simulink model "NeuralcircuitULInjured08102023_DSD"  (R2023a)
settings: Solver=VariableStepAuto  StartTime=0.0  StopTime=1600  RelTol=1e-3
values from neighbouring files (symbols this model uses):
  Cn = 1    [Inhibitory_excitatory_ULInjury_1Hz_08102023.m]    (also in Inhibitory_excitatory_ULInjury_30Hz_08102023.m; InitialExcitatoryInhibitoryNeurons_Healthy08062023.m; InitialExcitatoryInhibitoryULInjured_08102023_DSD.m)
  EK = -84*1    (= -84)    [Inhibitory_excitatory_ULInjury_1Hz_08102023.m]    (also in Inhibitory_excitatory_ULInjury_30Hz_08102023.m; InitialExcitatoryInhibitoryNeurons_Healthy08062023.m; InitialExcitatoryInhibitoryULInjured_08102023_DSD.m)
  EKEx = -90    [Inhibitory_excitatory_ULInjury_1Hz_08102023.m]    (also in Inhibitory_excitatory_ULInjury_30Hz_08102023.m; InitialExcitatoryInhibitoryNeurons_Healthy08062023.m; InitialExcitatoryInhibitoryULInjured_08102023_DSD.m)
  EKIn = -90    [Inhibitory_excitatory_ULInjury_1Hz_08102023.m]    (also in Inhibitory_excitatory_ULInjury_30Hz_08102023.m; InitialExcitatoryInhibitoryNeurons_Healthy08062023.m; InitialExcitatoryInhibitoryULInjured_08102023_DSD.m)
  ELEx = -65    [Inhibitory_excitatory_ULInjury_1Hz_08102023.m]    (also in Inhibitory_excitatory_ULInjury_30Hz_08102023.m; InitialExcitatoryInhibitoryNeurons_Healthy08062023.m; InitialExcitatoryInhibitoryULInjured_08102023_DSD.m)
  ELIn = -65    [Inhibitory_excitatory_ULInjury_1Hz_08102023.m]    (also in Inhibitory_excitatory_ULInjury_30Hz_08102023.m; InitialExcitatoryInhibitoryNeurons_Healthy08062023.m; InitialExcitatoryInhibitoryULInjured_08102023_DSD.m)
  ELk = -83.38*1    (= -83.38)    [Inhibitory_excitatory_ULInjury_1Hz_08102023.m]    (also in Inhibitory_excitatory_ULInjury_30Hz_08102023.m; InitialExcitatoryInhibitoryNeurons_Healthy08062023.m; InitialExcitatoryInhibitoryULInjured_08102023_DSD.m)
  ENa = 50*1    (= 50)    [Inhibitory_excitatory_ULInjury_1Hz_08102023.m]    (also in Inhibitory_excitatory_ULInjury_30Hz_08102023.m; InitialExcitatoryInhibitoryNeurons_Healthy08062023.m; InitialExcitatoryInhibitoryULInjured_08102023_DSD.m)
  ENaEx = 60    [Inhibitory_excitatory_ULInjury_1Hz_08102023.m]    (also in Inhibitory_excitatory_ULInjury_30Hz_08102023.m; InitialExcitatoryInhibitoryNeurons_Healthy08062023.m; InitialExcitatoryInhibitoryULInjured_08102023_DSD.m)
  ENaIn = 55    [Inhibitory_excitatory_ULInjury_1Hz_08102023.m]    (also in Inhibitory_excitatory_ULInjury_30Hz_08102023.m; InitialExcitatoryInhibitoryNeurons_Healthy08062023.m; InitialExcitatoryInhibitoryULInjured_08102023_DSD.m)
  ErestE = -65    [Inhibitory_excitatory_ULInjury_1Hz_08102023.m]    (also in Inhibitory_excitatory_ULInjury_30Hz_08102023.m; InitialExcitatoryInhibitoryNeurons_Healthy08062023.m; InitialExcitatoryInhibitoryULInjured_08102023_DSD.m)
  ErestIn = -64    [Inhibitory_excitatory_ULInjury_1Hz_08102023.m]    (also in Inhibitory_excitatory_ULInjury_30Hz_08102023.m; InitialExcitatoryInhibitoryNeurons_Healthy08062023.m; InitialExcitatoryInhibitoryULInjured_08102023_DSD.m)
  ESynE = -10    [Inhibitory_excitatory_ULInjury_1Hz_08102023.m]    (also in Inhibitory_excitatory_ULInjury_30Hz_08102023.m; InitialExcitatoryInhibitoryNeurons_Healthy08062023.m; InitialExcitatoryInhibitoryULInjured_08102023_DSD.m)
  ESynE2 = -10    [Inhibitory_excitatory_ULInjury_1Hz_08102023.m]    (also in Inhibitory_excitatory_ULInjury_30Hz_08102023.m; InitialExcitatoryInhibitoryNeurons_Healthy08062023.m; InitialExcitatoryInhibitoryULInjured_08102023_DSD.m)
  ESynE3 = -10    [Inhibitory_excitatory_ULInjury_1Hz_08102023.m]    (also in Inhibitory_excitatory_ULInjury_30Hz_08102023.m; InitialExcitatoryInhibitoryNeurons_Healthy08062023.m; InitialExcitatoryInhibitoryULInjured_08102023_DSD.m)
  ESynE4 = -10    [Inhibitory_excitatory_ULInjury_1Hz_08102023.m]    (also in Inhibitory_excitatory_ULInjury_30Hz_08102023.m; InitialExcitatoryInhibitoryNeurons_Healthy08062023.m; InitialExcitatoryInhibitoryULInjured_08102023_DSD.m)
  ESynE5 = -10    [Inhibitory_excitatory_ULInjury_1Hz_08102023.m]    (also in Inhibitory_excitatory_ULInjury_30Hz_08102023.m; InitialExcitatoryInhibitoryNeurons_Healthy08062023.m; InitialExcitatoryInhibitoryULInjured_08102023_DSD.m)
  ESynE6 = -15    [Inhibitory_excitatory_ULInjury_1Hz_08102023.m]    (also in Inhibitory_excitatory_ULInjury_30Hz_08102023.m; InitialExcitatoryInhibitoryNeurons_Healthy08062023.m; InitialExcitatoryInhibitoryULInjured_08102023_DSD.m = -10)
  ESynE7 = -10    [Inhibitory_excitatory_ULInjury_1Hz_08102023.m]    (also in Inhibitory_excitatory_ULInjury_30Hz_08102023.m; InitialExcitatoryInhibitoryNeurons_Healthy08062023.m; InitialExcitatoryInhibitoryULInjured_08102023_DSD.m)
  ESynI = -80    [Inhibitory_excitatory_ULInjury_1Hz_08102023.m]    (also in Inhibitory_excitatory_ULInjury_30Hz_08102023.m; InitialExcitatoryInhibitoryNeurons_Healthy08062023.m; InitialExcitatoryInhibitoryULInjured_08102023_DSD.m)
  ESynI2 = -80    [Inhibitory_excitatory_ULInjury_1Hz_08102023.m]    (also in Inhibitory_excitatory_ULInjury_30Hz_08102023.m; InitialExcitatoryInhibitoryNeurons_Healthy08062023.m; InitialExcitatoryInhibitoryULInjured_08102023_DSD.m)
  ESynI3 = -80    [Inhibitory_excitatory_ULInjury_1Hz_08102023.m]    (also in Inhibitory_excitatory_ULInjury_30Hz_08102023.m; InitialExcitatoryInhibitoryNeurons_Healthy08062023.m; InitialExcitatoryInhibitoryULInjured_08102023_DSD.m)
  ESynI5 = -80    [Inhibitory_excitatory_ULInjury_1Hz_08102023.m]    (also in Inhibitory_excitatory_ULInjury_30Hz_08102023.m; InitialExcitatoryInhibitoryNeurons_Healthy08062023.m; InitialExcitatoryInhibitoryULInjured_08102023_DSD.m)
  ESynI6 = -65    [Inhibitory_excitatory_ULInjury_1Hz_08102023.m]    (also in Inhibitory_excitatory_ULInjury_30Hz_08102023.m; InitialExcitatoryInhibitoryNeurons_Healthy08062023.m; InitialExcitatoryInhibitoryULInjured_08102023_DSD.m = -80)
  Exh0 = ahEx(V0)./(ahEx(V0)+bhEx(V0))    [Inhibitory_excitatory_ULInjury_1Hz_08102023.m]    (also in Inhibitory_excitatory_ULInjury_30Hz_08102023.m; InitialExcitatoryInhibitoryNeurons_Healthy08062023.m; InitialExcitatoryInhibitoryULInjured_08102023_DSD.m)
  Exm0 = amEx(V0)./(amEx(V0)+bmEx(V0))    [Inhibitory_excitatory_ULInjury_1Hz_08102023.m]    (also in Inhibitory_excitatory_ULInjury_30Hz_08102023.m; InitialExcitatoryInhibitoryNeurons_Healthy08062023.m; InitialExcitatoryInhibitoryULInjured_08102023_DSD.m)
  Exn0 = anEx(V0)./(anEx(V0)+bnEx(V0))    [Inhibitory_excitatory_ULInjury_1Hz_08102023.m]    (also in Inhibitory_excitatory_ULInjury_30Hz_08102023.m; InitialExcitatoryInhibitoryNeurons_Healthy08062023.m; InitialExcitatoryInhibitoryULInjured_08102023_DSD.m)
  Ga = 1*Gaxial    (= 0.351233961271)    [Inhibitory_excitatory_ULInjury_1Hz_08102023.m]    (also in Inhibitory_excitatory_ULInjury_30Hz_08102023.m; InitialExcitatoryInhibitoryNeurons_Healthy08062023.m; InitialExcitatoryInhibitoryULInjured_08102023_DSD.m)
  Gaxial = pi*(d^2)/(4*Ro_ax*Internodal_L)*1e7    (= 0.351233961271)    [Inhibitory_excitatory_ULInjury_1Hz_08102023.m]    (also in Inhibitory_excitatory_ULInjury_30Hz_08102023.m; InitialExcitatoryInhibitoryNeurons_Healthy08062023.m; InitialExcitatoryInhibitoryULInjured_08102023_DSD.m)
  gKEx = 100    [Inhibitory_excitatory_ULInjury_1Hz_08102023.m]    (also in Inhibitory_excitatory_ULInjury_30Hz_08102023.m; InitialExcitatoryInhibitoryNeurons_Healthy08062023.m; InitialExcitatoryInhibitoryULInjured_08102023_DSD.m)
  gKIn = 9    [Inhibitory_excitatory_ULInjury_1Hz_08102023.m]    (also in Inhibitory_excitatory_ULInjury_30Hz_08102023.m; InitialExcitatoryInhibitoryNeurons_Healthy08062023.m; InitialExcitatoryInhibitoryULInjured_08102023_DSD.m)
  gKs = 10*0.08/1    (= 0.8)    [Inhibitory_excitatory_ULInjury_1Hz_08102023.m]    (also in Inhibitory_excitatory_ULInjury_30Hz_08102023.m; InitialExcitatoryInhibitoryNeurons_Healthy08062023.m; InitialExcitatoryInhibitoryULInjured_08102023_DSD.m)
  gLEx = 0.1    [Inhibitory_excitatory_ULInjury_1Hz_08102023.m]    (also in Inhibitory_excitatory_ULInjury_30Hz_08102023.m; InitialExcitatoryInhibitoryNeurons_Healthy08062023.m; InitialExcitatoryInhibitoryULInjured_08102023_DSD.m)
  gLIn = 0.1    [Inhibitory_excitatory_ULInjury_1Hz_08102023.m]    (also in Inhibitory_excitatory_ULInjury_30Hz_08102023.m; InitialExcitatoryInhibitoryNeurons_Healthy08062023.m; InitialExcitatoryInhibitoryULInjured_08102023_DSD.m)
  gLk = 10*0.08/1    (= 0.8)    [Inhibitory_excitatory_ULInjury_1Hz_08102023.m]    (also in Inhibitory_excitatory_ULInjury_30Hz_08102023.m; InitialExcitatoryInhibitoryNeurons_Healthy08062023.m; InitialExcitatoryInhibitoryULInjured_08102023_DSD.m)
  gNaEx = 30    [Inhibitory_excitatory_ULInjury_1Hz_08102023.m]    (also in Inhibitory_excitatory_ULInjury_30Hz_08102023.m; InitialExcitatoryInhibitoryNeurons_Healthy08062023.m; InitialExcitatoryInhibitoryULInjured_08102023_DSD.m)
  gNaf = 10*3/1    (= 30)    [Inhibitory_excitatory_ULInjury_1Hz_08102023.m]    (also in Inhibitory_excitatory_ULInjury_30Hz_08102023.m; InitialExcitatoryInhibitoryNeurons_Healthy08062023.m; InitialExcitatoryInhibitoryULInjured_08102023_DSD.m)
  gNaIn = 35    [Inhibitory_excitatory_ULInjury_1Hz_08102023.m]    (also in Inhibitory_excitatory_ULInjury_30Hz_08102023.m; InitialExcitatoryInhibitoryNeurons_Healthy08062023.m; InitialExcitatoryInhibitoryULInjured_08102023_DSD.m)
  gNap = 10*0.005/1    (= 0.05)    [Inhibitory_excitatory_ULInjury_1Hz_08102023.m]    (also in Inhibitory_excitatory_ULInjury_30Hz_08102023.m; InitialExcitatoryInhibitoryNeurons_Healthy08062023.m; InitialExcitatoryInhibitoryULInjured_08102023_DSD.m)
  gSynE = 0.08    [Inhibitory_excitatory_ULInjury_1Hz_08102023.m]    (also in Inhibitory_excitatory_ULInjury_30Hz_08102023.m; InitialExcitatoryInhibitoryNeurons_Healthy08062023.m; InitialExcitatoryInhibitoryULInjured_08102023_DSD.m)
  gSynE2 = 0.08    [Inhibitory_excitatory_ULInjury_1Hz_08102023.m]    (also in Inhibitory_excitatory_ULInjury_30Hz_08102023.m; InitialExcitatoryInhibitoryNeurons_Healthy08062023.m; InitialExcitatoryInhibitoryULInjured_08102023_DSD.m)
  gSynE3 = 0.08    [Inhibitory_excitatory_ULInjury_1Hz_08102023.m]    (also in Inhibitory_excitatory_ULInjury_30Hz_08102023.m; InitialExcitatoryInhibitoryNeurons_Healthy08062023.m; InitialExcitatoryInhibitoryULInjured_08102023_DSD.m)
  gSynE4 = 0.08    [Inhibitory_excitatory_ULInjury_1Hz_08102023.m]    (also in Inhibitory_excitatory_ULInjury_30Hz_08102023.m; InitialExcitatoryInhibitoryNeurons_Healthy08062023.m; InitialExcitatoryInhibitoryULInjured_08102023_DSD.m)
  gSynE5 = 0.08    [Inhibitory_excitatory_ULInjury_1Hz_08102023.m]    (also in Inhibitory_excitatory_ULInjury_30Hz_08102023.m; InitialExcitatoryInhibitoryNeurons_Healthy08062023.m; InitialExcitatoryInhibitoryULInjured_08102023_DSD.m)
  gSynE6 = 0.08    [Inhibitory_excitatory_ULInjury_1Hz_08102023.m]    (also in Inhibitory_excitatory_ULInjury_30Hz_08102023.m; InitialExcitatoryInhibitoryNeurons_Healthy08062023.m; InitialExcitatoryInhibitoryULInjured_08102023_DSD.m)
  gSynE7 = 0.165    [Inhibitory_excitatory_ULInjury_1Hz_08102023.m]    (also in Inhibitory_excitatory_ULInjury_30Hz_08102023.m; InitialExcitatoryInhibitoryNeurons_Healthy08062023.m; InitialExcitatoryInhibitoryULInjured_08102023_DSD.m)
  gSynI = 0.8    [Inhibitory_excitatory_ULInjury_1Hz_08102023.m]    (also in Inhibitory_excitatory_ULInjury_30Hz_08102023.m; InitialExcitatoryInhibitoryNeurons_Healthy08062023.m; InitialExcitatoryInhibitoryULInjured_08102023_DSD.m)
  gSynI2 = 0.12    [Inhibitory_excitatory_ULInjury_1Hz_08102023.m]    (also in Inhibitory_excitatory_ULInjury_30Hz_08102023.m; InitialExcitatoryInhibitoryNeurons_Healthy08062023.m; InitialExcitatoryInhibitoryULInjured_08102023_DSD.m)
  gSynI3 = 0.12    [Inhibitory_excitatory_ULInjury_1Hz_08102023.m]    (also in Inhibitory_excitatory_ULInjury_30Hz_08102023.m; InitialExcitatoryInhibitoryNeurons_Healthy08062023.m; InitialExcitatoryInhibitoryULInjured_08102023_DSD.m)
  gSynI5 = 0.12    [Inhibitory_excitatory_ULInjury_1Hz_08102023.m]    (also in Inhibitory_excitatory_ULInjury_30Hz_08102023.m; InitialExcitatoryInhibitoryNeurons_Healthy08062023.m; InitialExcitatoryInhibitoryULInjured_08102023_DSD.m)
  gSynI6 = 0.12    [Inhibitory_excitatory_ULInjury_1Hz_08102023.m]    (also in Inhibitory_excitatory_ULInjury_30Hz_08102023.m; InitialExcitatoryInhibitoryNeurons_Healthy08062023.m; InitialExcitatoryInhibitoryULInjured_08102023_DSD.m)
  h0 = ah(V0O)./(ah(V0O)+bh(V0O))    [Inhibitory_excitatory_ULInjury_1Hz_08102023.m]    (also in Inhibitory_excitatory_ULInjury_30Hz_08102023.m; InitialExcitatoryInhibitoryNeurons_Healthy08062023.m; InitialExcitatoryInhibitoryULInjured_08102023_DSD.m)
  Inh0 = ahIn(ErestIn)./(ahIn(ErestIn)+bhIn(ErestIn))    [Inhibitory_excitatory_ULInjury_1Hz_08102023.m]    (also in Inhibitory_excitatory_ULInjury_30Hz_08102023.m; InitialExcitatoryInhibitoryNeurons_Healthy08062023.m; InitialExcitatoryInhibitoryULInjured_08102023_DSD.m)
  Inm0 = amIn(ErestIn)./(amIn(ErestIn)+bmIn(ErestIn))    [Inhibitory_excitatory_ULInjury_1Hz_08102023.m]    (also in Inhibitory_excitatory_ULInjury_30Hz_08102023.m; InitialExcitatoryInhibitoryNeurons_Healthy08062023.m; InitialExcitatoryInhibitoryULInjured_08102023_DSD.m)
  Inn0 = anIn(ErestIn)./(anIn(ErestIn)+bnIn(ErestIn))    [Inhibitory_excitatory_ULInjury_1Hz_08102023.m]    (also in Inhibitory_excitatory_ULInjury_30Hz_08102023.m; InitialExcitatoryInhibitoryNeurons_Healthy08062023.m; InitialExcitatoryInhibitoryULInjured_08102023_DSD.m)
  m0 = am(V0O)./(am(V0O)+Bm(V0O))    [Inhibitory_excitatory_ULInjury_1Hz_08102023.m]    (also in Inhibitory_excitatory_ULInjury_30Hz_08102023.m; InitialExcitatoryInhibitoryNeurons_Healthy08062023.m; InitialExcitatoryInhibitoryULInjured_08102023_DSD.m)
  mNap0 = amNap(V0)./(amNap(V0O)+bmNap(V0O))    [Inhibitory_excitatory_ULInjury_1Hz_08102023.m]    (also in Inhibitory_excitatory_ULInjury_30Hz_08102023.m; InitialExcitatoryInhibitoryNeurons_Healthy08062023.m; InitialExcitatoryInhibitoryULInjured_08102023_DSD.m)
  Ro_e = 500    [Inhibitory_excitatory_ULInjury_1Hz_08102023.m]    (also in Inhibitory_excitatory_ULInjury_30Hz_08102023.m; InitialExcitatoryInhibitoryNeurons_Healthy08062023.m; InitialExcitatoryInhibitoryULInjured_08102023_DSD.m)
  s0 = as(V0O)./(as(V0O)+bs(V0O))    [Inhibitory_excitatory_ULInjury_1Hz_08102023.m]    (also in Inhibitory_excitatory_ULInjury_30Hz_08102023.m; InitialExcitatoryInhibitoryNeurons_Healthy08062023.m; InitialExcitatoryInhibitoryULInjured_08102023_DSD.m)
  TawIExt = 30    [Inhibitory_excitatory_ULInjury_1Hz_08102023.m]    (also in Inhibitory_excitatory_ULInjury_30Hz_08102023.m; InitialExcitatoryInhibitoryNeurons_Healthy08062023.m = 200; InitialExcitatoryInhibitoryULInjured_08102023_DSD.m = 200)
  TawIExtE = 30    [Inhibitory_excitatory_ULInjury_1Hz_08102023.m]    (also in Inhibitory_excitatory_ULInjury_30Hz_08102023.m; InitialExcitatoryInhibitoryNeurons_Healthy08062023.m = 1; InitialExcitatoryInhibitoryULInjured_08102023_DSD.m = 10)
  TawSynE = 5    [Inhibitory_excitatory_ULInjury_1Hz_08102023.m]    (also in Inhibitory_excitatory_ULInjury_30Hz_08102023.m; InitialExcitatoryInhibitoryNeurons_Healthy08062023.m; InitialExcitatoryInhibitoryULInjured_08102023_DSD.m)
  TawSynE2 = 11    [Inhibitory_excitatory_ULInjury_1Hz_08102023.m]    (also in Inhibitory_excitatory_ULInjury_30Hz_08102023.m; InitialExcitatoryInhibitoryNeurons_Healthy08062023.m = 12; InitialExcitatoryInhibitoryULInjured_08102023_DSD.m = 5)
  TawSynE3 = 10    [Inhibitory_excitatory_ULInjury_1Hz_08102023.m]    (also in Inhibitory_excitatory_ULInjury_30Hz_08102023.m; InitialExcitatoryInhibitoryNeurons_Healthy08062023.m = 18; InitialExcitatoryInhibitoryULInjured_08102023_DSD.m = 8)
  TawSynE4 = 6    [Inhibitory_excitatory_ULInjury_1Hz_08102023.m]    (also in Inhibitory_excitatory_ULInjury_30Hz_08102023.m; InitialExcitatoryInhibitoryNeurons_Healthy08062023.m; InitialExcitatoryInhibitoryULInjured_08102023_DSD.m)
  TawSynE41 = 14    [Inhibitory_excitatory_ULInjury_1Hz_08102023.m]    (also in Inhibitory_excitatory_ULInjury_30Hz_08102023.m; InitialExcitatoryInhibitoryNeurons_Healthy08062023.m = 15; InitialExcitatoryInhibitoryULInjured_08102023_DSD.m = 6)
  TawSynE5 = 6    [Inhibitory_excitatory_ULInjury_1Hz_08102023.m]    (also in Inhibitory_excitatory_ULInjury_30Hz_08102023.m; InitialExcitatoryInhibitoryNeurons_Healthy08062023.m; InitialExcitatoryInhibitoryULInjured_08102023_DSD.m)
  TawSynE6 = 3    [Inhibitory_excitatory_ULInjury_1Hz_08102023.m]    (also in Inhibitory_excitatory_ULInjury_30Hz_08102023.m; InitialExcitatoryInhibitoryNeurons_Healthy08062023.m; InitialExcitatoryInhibitoryULInjured_08102023_DSD.m)
  TawSynE66 = 1    [Inhibitory_excitatory_ULInjury_1Hz_08102023.m]    (also in Inhibitory_excitatory_ULInjury_30Hz_08102023.m; InitialExcitatoryInhibitoryNeurons_Healthy08062023.m; InitialExcitatoryInhibitoryULInjured_08102023_DSD.m)
  TawSynE66E = 5    [Inhibitory_excitatory_ULInjury_1Hz_08102023.m]    (also in Inhibitory_excitatory_ULInjury_30Hz_08102023.m; InitialExcitatoryInhibitoryNeurons_Healthy08062023.m; InitialExcitatoryInhibitoryULInjured_08102023_DSD.m)
  TawSynE7 = 0.05    [Inhibitory_excitatory_ULInjury_1Hz_08102023.m]    (also in Inhibitory_excitatory_ULInjury_30Hz_08102023.m; InitialExcitatoryInhibitoryNeurons_Healthy08062023.m; InitialExcitatoryInhibitoryULInjured_08102023_DSD.m)
  TawSynI = 5    [Inhibitory_excitatory_ULInjury_1Hz_08102023.m]    (also in Inhibitory_excitatory_ULInjury_30Hz_08102023.m; InitialExcitatoryInhibitoryNeurons_Healthy08062023.m; InitialExcitatoryInhibitoryULInjured_08102023_DSD.m)
  TawSynI2 = 1    [Inhibitory_excitatory_ULInjury_1Hz_08102023.m]    (also in Inhibitory_excitatory_ULInjury_30Hz_08102023.m; InitialExcitatoryInhibitoryNeurons_Healthy08062023.m; InitialExcitatoryInhibitoryULInjured_08102023_DSD.m = 2)
  TawSynI3 = 30    [Inhibitory_excitatory_ULInjury_1Hz_08102023.m]    (also in Inhibitory_excitatory_ULInjury_30Hz_08102023.m; InitialExcitatoryInhibitoryNeurons_Healthy08062023.m = 35; InitialExcitatoryInhibitoryULInjured_08102023_DSD.m)
  TawSynI5 = 4    [Inhibitory_excitatory_ULInjury_1Hz_08102023.m]    (also in Inhibitory_excitatory_ULInjury_30Hz_08102023.m; InitialExcitatoryInhibitoryNeurons_Healthy08062023.m = 1; InitialExcitatoryInhibitoryULInjured_08102023_DSD.m = 1)
  TawSynI6 = 3    [Inhibitory_excitatory_ULInjury_1Hz_08102023.m]    (also in Inhibitory_excitatory_ULInjury_30Hz_08102023.m; InitialExcitatoryInhibitoryNeurons_Healthy08062023.m; InitialExcitatoryInhibitoryULInjured_08102023_DSD.m)
  TawSynI7 = 0.01    [Inhibitory_excitatory_ULInjury_1Hz_08102023.m]    (also in Inhibitory_excitatory_ULInjury_30Hz_08102023.m; InitialExcitatoryInhibitoryNeurons_Healthy08062023.m; InitialExcitatoryInhibitoryULInjured_08102023_DSD.m)
  V0 = -65    [Inhibitory_excitatory_ULInjury_1Hz_08102023.m]    (also in Inhibitory_excitatory_ULInjury_30Hz_08102023.m; InitialExcitatoryInhibitoryNeurons_Healthy08062023.m; InitialExcitatoryInhibitoryULInjured_08102023_DSD.m)
  V0In = -64    [Inhibitory_excitatory_ULInjury_1Hz_08102023.m]    (also in Inhibitory_excitatory_ULInjury_30Hz_08102023.m; InitialExcitatoryInhibitoryNeurons_Healthy08062023.m; InitialExcitatoryInhibitoryULInjured_08102023_DSD.m)
  w12 = -0.2    [Inhibitory_excitatory_ULInjury_1Hz_08102023.m]    (also in Inhibitory_excitatory_ULInjury_30Hz_08102023.m; InitialExcitatoryInhibitoryNeurons_Healthy08062023.m = -0.28; InitialExcitatoryInhibitoryULInjured_08102023_DSD.m = -0.35)
  w14 = 0.05    [Inhibitory_excitatory_ULInjury_1Hz_08102023.m]    (also in Inhibitory_excitatory_ULInjury_30Hz_08102023.m; InitialExcitatoryInhibitoryNeurons_Healthy08062023.m = 0.09; InitialExcitatoryInhibitoryULInjured_08102023_DSD.m = 0.09)
  w15 = -0.45    [Inhibitory_excitatory_ULInjury_1Hz_08102023.m]    (also in Inhibitory_excitatory_ULInjury_30Hz_08102023.m = -0.07; InitialExcitatoryInhibitoryNeurons_Healthy08062023.m = -0.4; InitialExcitatoryInhibitoryULInjured_08102023_DSD.m = -0.4)
  w17 = -0.25    [Inhibitory_excitatory_ULInjury_1Hz_08102023.m]    (also in Inhibitory_excitatory_ULInjury_30Hz_08102023.m; InitialExcitatoryInhibitoryNeurons_Healthy08062023.m; InitialExcitatoryInhibitoryULInjured_08102023_DSD.m)
  w26 = 0.2    [Inhibitory_excitatory_ULInjury_1Hz_08102023.m]    (also in Inhibitory_excitatory_ULInjury_30Hz_08102023.m = 0.25; InitialExcitatoryInhibitoryNeurons_Healthy08062023.m = 0.05; InitialExcitatoryInhibitoryULInjured_08102023_DSD.m = 0.05)
  w28 = 0.165    [Inhibitory_excitatory_ULInjury_1Hz_08102023.m]    (also in Inhibitory_excitatory_ULInjury_30Hz_08102023.m; InitialExcitatoryInhibitoryNeurons_Healthy08062023.m = 0.13; InitialExcitatoryInhibitoryULInjured_08102023_DSD.m = 0.13)
  w34 = 0.09    [Inhibitory_excitatory_ULInjury_1Hz_08102023.m]    (also in Inhibitory_excitatory_ULInjury_30Hz_08102023.m; InitialExcitatoryInhibitoryNeurons_Healthy08062023.m = 0.03; InitialExcitatoryInhibitoryULInjured_08102023_DSD.m = 0.06)
  w63 = -0.12    [Inhibitory_excitatory_ULInjury_1Hz_08102023.m]    (also in Inhibitory_excitatory_ULInjury_30Hz_08102023.m; InitialExcitatoryInhibitoryNeurons_Healthy08062023.m = -0.08; InitialExcitatoryInhibitoryULInjured_08102023_DSD.m = -0.27)
  w66 = 0.03    [Inhibitory_excitatory_ULInjury_1Hz_08102023.m]    (also in Inhibitory_excitatory_ULInjury_30Hz_08102023.m; InitialExcitatoryInhibitoryNeurons_Healthy08062023.m; InitialExcitatoryInhibitoryULInjured_08102023_DSD.m)
  w66E = 0.2    [Inhibitory_excitatory_ULInjury_1Hz_08102023.m]    (also in Inhibitory_excitatory_ULInjury_30Hz_08102023.m; InitialExcitatoryInhibitoryNeurons_Healthy08062023.m = 0.09; InitialExcitatoryInhibitoryULInjured_08102023_DSD.m = 0.1)
  w67 = -0.4    [Inhibitory_excitatory_ULInjury_1Hz_08102023.m]    (also in Inhibitory_excitatory_ULInjury_30Hz_08102023.m; InitialExcitatoryInhibitoryNeurons_Healthy08062023.m = -0.55; InitialExcitatoryInhibitoryULInjured_08102023_DSD.m = -0.55)
  w68 = 0.35    [Inhibitory_excitatory_ULInjury_1Hz_08102023.m]    (also in Inhibitory_excitatory_ULInjury_30Hz_08102023.m; InitialExcitatoryInhibitoryNeurons_Healthy08062023.m = 0.1; InitialExcitatoryInhibitoryULInjured_08102023_DSD.m = 0.1)
  w71 = 0.25    [Inhibitory_excitatory_ULInjury_1Hz_08102023.m]    (also in Inhibitory_excitatory_ULInjury_30Hz_08102023.m; InitialExcitatoryInhibitoryNeurons_Healthy08062023.m; InitialExcitatoryInhibitoryULInjured_08102023_DSD.m)
  w78 = 0.25    [Inhibitory_excitatory_ULInjury_1Hz_08102023.m]    (also in Inhibitory_excitatory_ULInjury_30Hz_08102023.m; InitialExcitatoryInhibitoryNeurons_Healthy08062023.m; InitialExcitatoryInhibitoryULInjured_08102023_DSD.m)
  w79 = 0.35    [Inhibitory_excitatory_ULInjury_1Hz_08102023.m]    (also in Inhibitory_excitatory_ULInjury_30Hz_08102023.m; InitialExcitatoryInhibitoryNeurons_Healthy08062023.m; InitialExcitatoryInhibitoryULInjured_08102023_DSD.m)
  w83 = 0.2    [Inhibitory_excitatory_ULInjury_1Hz_08102023.m]    (also in Inhibitory_excitatory_ULInjury_30Hz_08102023.m; InitialExcitatoryInhibitoryNeurons_Healthy08062023.m = 0.13; InitialExcitatoryInhibitoryULInjured_08102023_DSD.m = 0.08)
  w85 = 0.1    [Inhibitory_excitatory_ULInjury_1Hz_08102023.m]    (also in Inhibitory_excitatory_ULInjury_30Hz_08102023.m = 0.12; InitialExcitatoryInhibitoryNeurons_Healthy08062023.m = 0.04; InitialExcitatoryInhibitoryULInjured_08102023_DSD.m = 0.05)
  X = nan(node,1)    [Inhibitory_excitatory_ULInjury_1Hz_08102023.m]    (also in Inhibitory_excitatory_ULInjury_30Hz_08102023.m; InitialExcitatoryInhibitoryNeurons_Healthy08062023.m; InitialExcitatoryInhibitoryULInjured_08102023_DSD.m)
  X2 = nan(node2,1)    [Inhibitory_excitatory_ULInjury_1Hz_08102023.m]    (also in Inhibitory_excitatory_ULInjury_30Hz_08102023.m; InitialExcitatoryInhibitoryNeurons_Healthy08062023.m; InitialExcitatoryInhibitoryULInjured_08102023_DSD.m)
  Xelec = Xtotal-Nodal_L*9-Internodal_L*9    (= 0.1152)    [Inhibitory_excitatory_ULInjury_1Hz_08102023.m]    (also in Inhibitory_excitatory_ULInjury_30Hz_08102023.m; InitialExcitatoryInhibitoryNeurons_Healthy08062023.m; InitialExcitatoryInhibitoryULInjured_08102023_DSD.m)
  Xelec2 = 1/(10000)+Nodal_L2*(node2-1)/2+Internodal_L2*(node2-1)/2    (= 0.0001)    [Inhibitory_excitatory_ULInjury_1Hz_08102023.m]    (also in Inhibitory_excitatory_ULInjury_30Hz_08102023.m; InitialExcitatoryInhibitoryNeurons_Healthy08062023.m; InitialExcitatoryInhibitoryULInjured_08102023_DSD.m)
  Y = nan(node,1)    [Inhibitory_excitatory_ULInjury_1Hz_08102023.m]    (also in Inhibitory_excitatory_ULInjury_30Hz_08102023.m; InitialExcitatoryInhibitoryNeurons_Healthy08062023.m; InitialExcitatoryInhibitoryULInjured_08102023_DSD.m)
  Y2 = nan(node2,1)    [Inhibitory_excitatory_ULInjury_1Hz_08102023.m]    (also in Inhibitory_excitatory_ULInjury_30Hz_08102023.m; InitialExcitatoryInhibitoryNeurons_Healthy08062023.m; InitialExcitatoryInhibitoryULInjured_08102023_DSD.m)
  Yelec = 100/10000    (= 0.01)    [Inhibitory_excitatory_ULInjury_1Hz_08102023.m]    (also in Inhibitory_excitatory_ULInjury_30Hz_08102023.m; InitialExcitatoryInhibitoryNeurons_Healthy08062023.m; InitialExcitatoryInhibitoryULInjured_08102023_DSD.m)
  Yelec2 = 500/10000    (= 0.05)    [Inhibitory_excitatory_ULInjury_1Hz_08102023.m]    (also in Inhibitory_excitatory_ULInjury_30Hz_08102023.m; InitialExcitatoryInhibitoryNeurons_Healthy08062023.m; InitialExcitatoryInhibitoryULInjured_08102023_DSD.m)
libraries: simulink x1
(part 13 of 14)

== system NeuralcircuitULInjured08102023_DSD/Neuron 8/Node 6/Naf/h ==
  Vi : Inport
  Add : Sum  Inputs=+-
  Add1 : Sum
  Add2 : Sum  Inputs=+-
  Add3 : Sum  Inputs=+-
  Add4 : Sum
  Add5 : Sum
  Beta_h : Product  Inputs=*/
  Constant : Constant
  Constant1 : Constant  Value=0.0336
  Constant10 : Constant  Value=13.4
  Constant2 : Constant  Value=118
  Constant3 : Constant
  Constant5 : Constant  Value=11
  Constant6 : Constant  Value=2.3
  Constant7 : Constant  Value=35.8
  Constant8 : Constant
  Divide : Product  Inputs=**
  Divide1 : Product  Inputs=**
  Divide4 : Product  Inputs=*/
  Divide5 : Product  Inputs=**
  Divide6 : Product  Inputs=*/
  Gain : Gain  Gain=-1
  Gain1 : Gain  Gain=-1
  Integrator Limited : Integrator  InitialCondition=h0  UpperSaturationLimit=1  LowerSaturationLimit=0
  Math Function : Math  SignedPower=on
  Math Function1 : Math  SignedPower=on
  alpha_h1 : Product  Inputs=*/
  hNaf : Outport  VectorParamsAs1DForOutWhenUnconnected=off
  wires:
  Add5/1 -> Beta_h/2
  Divide/1 -> Add3/1
  Constant6/1 -> Beta_h/1
  Divide5/1 -> Add3/2
  Add/1 -> Divide/1
  Constant/1 -> Add/1
  Add1/1 -> Divide4/1, Gain1/1
  Constant2/1 -> Add1/1
  Constant7/1 -> Add4/1
  Constant8/1 -> Add5/1
  Add4/1 -> Gain/1
  Divide6/1 -> Math Function1/1
  Math Function1/1 -> Add5/2
  Constant10/1 -> Divide6/2
  Constant1/1 -> Divide1/1
  Beta_h/1 -> Divide5/2
  Add3/1 -> Integrator Limited/1
  Divide4/1 -> Math Function/1
  Divide1/1 -> alpha_h1/1
  Vi/1 -> Add4/2, Add1/2
  Gain/1 -> Divide6/1
  Integrator Limited/1 -> hNaf/1, Add/2, Divide5/1
  Gain1/1 -> Divide1/2
  Constant5/1 -> Divide4/2
  Add2/1 -> alpha_h1/2
  Constant3/1 -> Add2/1
  Math Function/1 -> Add2/2
  alpha_h1/1 -> Divide/2

== system NeuralcircuitULInjured08102023_DSD/Neuron 8/Node 6/Naf/m  ==
  Vm : Inport
  Add{,2..3,5} (4 alike) : Sum  Inputs=+-
  Add1 : Sum
  Add4 : Sum
  Constant : Constant
  Constant1 : Constant  Value=1.86
  Constant10 : Constant  Value=9.16
  Constant2 : Constant  Value=25.4
  Constant3 : Constant
  Constant4 : Constant  Value=-1
  Constant5 : Constant  Value=10.3
  Constant6 : Constant  Value=0.086
  Constant7 : Constant  Value=29.7
  Constant8 : Constant
  Divide{,1..3,5} (5 alike) : Product  Inputs=**
  Divide4 : Product  Inputs=*/
  Divide6 : Product  Inputs=*/
  Gain : Gain  Gain=-1
  Integrator Limited : Integrator  InitialCondition=m0  UpperSaturationLimit=1  LowerSaturationLimit=0
  Math Function : Math  SignedPower=on
  Math Function1 : Math  SignedPower=on
  alpha_m : Product  Inputs=*/
  alpha_m1 : Product  Inputs=*/
  mNaf : Outport  VectorParamsAs1DForOutWhenUnconnected=off
  wires:
  Gain/1 -> Divide2/2
  Divide/1 -> Add3/1
  Divide5/1 -> Add3/2
  Add/1 -> Divide/1
  Constant/1 -> Add/1
  Divide3/1 -> Divide4/1
  Constant2/1 -> Add1/1
  Constant6/1 -> Divide2/1
  Constant7/1 -> Add4/1
  Add4/1 -> Divide6/1, Gain/1
  Divide6/1 -> Math Function1/1
  Constant10/1 -> Divide6/2
  Divide1/1 -> alpha_m/1
  Integrator Limited/1 -> mNaf/1, Add/2, Divide5/1
  Constant3/1 -> Add2/1
  Constant5/1 -> Divide4/2
  Add1/1 -> Divide3/1, Divide1/2
  Constant1/1 -> Divide1/1
  Add2/1 -> alpha_m/2
  Constant4/1 -> Divide3/2
  Add3/1 -> Integrator Limited/1
  Math Function/1 -> Add2/2
  Divide4/1 -> Math Function/1
  alpha_m/1 -> Divide/2
  Vm/1 -> Add4/2, Add1/2
  Constant8/1 -> Add5/1
  Math Function1/1 -> Add5/2
  Add5/1 -> alpha_m1/2
  alpha_m1/1 -> Divide5/2
  Divide2/1 -> alpha_m1/1

== system NeuralcircuitULInjured08102023_DSD/Neuron 8/Node 6/Naf1/m  ==
  Vm : Inport
  Add{,2..3,5} (4 alike) : Sum  Inputs=+-
  Add1 : Sum
  Add4 : Sum
  Constant : Constant
  Constant1 : Constant  Value=0.186
  Constant10 : Constant  Value=9.16
  Constant2 : Constant  Value=48.4
  Constant3 : Constant
  Constant4 : Constant  Value=-1
  Constant5 : Constant  Value=10.3
  Constant6 : Constant  Value=0.0086
  Constant7 : Constant  Value=42.7
  Constant8 : Constant
  Divide{,1..3,5} (5 alike) : Product  Inputs=**
  Divide4 : Product  Inputs=*/
  Divide6 : Product  Inputs=*/
  Gain : Gain  Gain=-1
  Integrator Limited : Integrator  InitialCondition=mNap0  UpperSaturationLimit=1  LowerSaturationLimit=0
  Math Function : Math  SignedPower=on
  Math Function1 : Math  SignedPower=on
  alpha_m : Product  Inputs=*/
  alpha_m1 : Product  Inputs=*/
  mNap : Outport  VectorParamsAs1DForOutWhenUnconnected=off
  wires:
  Divide/1 -> Add3/1
  Divide5/1 -> Add3/2
  Add/1 -> Divide/1
  Constant/1 -> Add/1
  Divide3/1 -> Divide4/1
  Constant2/1 -> Add1/1
  Constant6/1 -> Divide2/1
  Constant7/1 -> Add4/1
  Add4/1 -> Divide6/1, Gain/1
  Divide6/1 -> Math Function1/1
  Constant10/1 -> Divide6/2
  Divide1/1 -> alpha_m/1
  Integrator Limited/1 -> mNap/1, [mNap], Add/2, Divide5/1
  Constant3/1 -> Add2/1
  Constant5/1 -> Divide4/2
  Add1/1 -> Divide3/1, Divide1/2
  Constant1/1 -> Divide1/1
  Add2/1 -> alpha_m/2
  Constant4/1 -> Divide3/2
  Add3/1 -> Integrator Limited/1
  Math Function/1 -> Add2/2
  Divide4/1 -> Math Function/1
  alpha_m/1 -> Divide/2
  Vm/1 -> Add4/2, Add1/2
  alpha_m1/1 -> Divide5/2
  Divide2/1 -> alpha_m1/1
  Gain/1 -> Divide2/2
  Add5/1 -> alpha_m1/2
  Constant8/1 -> Add5/1
  Math Function1/1 -> Add5/2

== system NeuralcircuitULInjured08102023_DSD/Neuron 8/Node 7/Ks/s  ==
  Vm : Inport
  Add{,2..3,5} (4 alike) : Sum  Inputs=+-
  Add1 : Sum
  Add4 : Sum
  Beta_s : Product  Inputs=*/
  Constant : Constant
  Constant1 : Constant  Value=0.00122
  Constant10 : Constant  Value=21.8
  Constant2 : Constant  Value=19.5
  Constant3 : Constant
  Constant4 : Constant  Value=-1
  Constant5 : Constant  Value=23.6
  Constant6 : Constant  Value=0.000739
  Constant7 : Constant  Value=87.1
  Constant8 : Constant
  Divide{,1..3,5} (5 alike) : Product  Inputs=**
  Divide4 : Product  Inputs=*/
  Divide6 : Product  Inputs=*/
  Gain : Gain  Gain=-1
  Integrator Limited : Integrator  InitialCondition=s0  UpperSaturationLimit=1  LowerSaturationLimit=0
  Math Function : Math  SignedPower=on
  Math Function1 : Math  SignedPower=on
  alpha_m : Product  Inputs=*/
  s : Outport  VectorParamsAs1DForOutWhenUnconnected=off
  wires:
  Divide/1 -> Add3/1
  Divide5/1 -> Add3/2
  Add/1 -> Divide/1
  Constant/1 -> Add/1
  Divide3/1 -> Divide4/1
  Constant2/1 -> Add1/1
  Constant6/1 -> Divide2/1
  Constant7/1 -> Add4/1
  Add4/1 -> Divide6/1, Gain/1
  Divide6/1 -> Math Function1/1
  Constant10/1 -> Divide6/2
  Divide1/1 -> alpha_m/1
  Integrator Limited/1 -> Add/2, Divide5/1, s/1
  Constant3/1 -> Add2/1
  Constant5/1 -> Divide4/2
  Add1/1 -> Divide3/1, Divide1/2
  Constant1/1 -> Divide1/1
  Add2/1 -> alpha_m/2
  Constant4/1 -> Divide3/2
  Add3/1 -> Integrator Limited/1
  Math Function/1 -> Add2/2
  Divide4/1 -> Math Function/1
  alpha_m/1 -> Divide/2
  Vm/1 -> Add4/2, Add1/2
  Gain/1 -> Divide2/2
  Beta_s/1 -> Divide5/2
  Divide2/1 -> Beta_s/1
  Constant8/1 -> Add5/1
  Add5/1 -> Beta_s/2
  Math Function1/1 -> Add5/2

== system NeuralcircuitULInjured08102023_DSD/Neuron 8/Node 7/Naf/h ==
  Vi : Inport
  Add : Sum  Inputs=+-
  Add1 : Sum
  Add2 : Sum  Inputs=+-
  Add3 : Sum  Inputs=+-
  Add4 : Sum
  Add5 : Sum
  Beta_h : Product  Inputs=*/
  Constant : Constant
  Constant1 : Constant  Value=0.0336
  Constant10 : Constant  Value=13.4
  Constant2 : Constant  Value=118
  Constant3 : Constant
  Constant5 : Constant  Value=11
  Constant6 : Constant  Value=2.3
  Constant7 : Constant  Value=35.8
  Constant8 : Constant
  Divide : Product  Inputs=**
  Divide1 : Product  Inputs=**
  Divide4 : Product  Inputs=*/
  Divide5 : Product  Inputs=**
  Divide6 : Product  Inputs=*/
  Gain : Gain  Gain=-1
  Gain1 : Gain  Gain=-1
  Integrator Limited : Integrator  InitialCondition=h0  UpperSaturationLimit=1  LowerSaturationLimit=0
  Math Function : Math  SignedPower=on
  Math Function1 : Math  SignedPower=on
  alpha_h1 : Product  Inputs=*/
  hNaf : Outport  VectorParamsAs1DForOutWhenUnconnected=off
  wires:
  Add5/1 -> Beta_h/2
  Divide/1 -> Add3/1
  Constant6/1 -> Beta_h/1
  Divide5/1 -> Add3/2
  Add/1 -> Divide/1
  Constant/1 -> Add/1
  Add1/1 -> Divide4/1, Gain1/1
  Constant2/1 -> Add1/1
  Constant7/1 -> Add4/1
  Constant8/1 -> Add5/1
  Add4/1 -> Gain/1
  Divide6/1 -> Math Function1/1
  Math Function1/1 -> Add5/2
  Constant10/1 -> Divide6/2
  Constant1/1 -> Divide1/1
  Beta_h/1 -> Divide5/2
  Add3/1 -> Integrator Limited/1
  Divide4/1 -> Math Function/1
  Divide1/1 -> alpha_h1/1
  Vi/1 -> Add4/2, Add1/2
  Gain/1 -> Divide6/1
  Integrator Limited/1 -> hNaf/1, Add/2, Divide5/1
  Gain1/1 -> Divide1/2
  Constant5/1 -> Divide4/2
  Add2/1 -> alpha_h1/2
  Constant3/1 -> Add2/1
  Math Function/1 -> Add2/2
  alpha_h1/1 -> Divide/2

== system NeuralcircuitULInjured08102023_DSD/Neuron 8/Node 7/Naf/m  ==
  Vm : Inport
  Add{,2..3,5} (4 alike) : Sum  Inputs=+-
  Add1 : Sum
  Add4 : Sum
  Constant : Constant
  Constant1 : Constant  Value=1.86
  Constant10 : Constant  Value=9.16
  Constant2 : Constant  Value=25.4
  Constant3 : Constant
  Constant4 : Constant  Value=-1
  Constant5 : Constant  Value=10.3
  Constant6 : Constant  Value=0.086
  Constant7 : Constant  Value=29.7
  Constant8 : Constant
  Divide{,1..3,5} (5 alike) : Product  Inputs=**
  Divide4 : Product  Inputs=*/
  Divide6 : Product  Inputs=*/
  Gain : Gain  Gain=-1
  Integrator Limited : Integrator  InitialCondition=m0  UpperSaturationLimit=1  LowerSaturationLimit=0
  Math Function : Math  SignedPower=on
  Math Function1 : Math  SignedPower=on
  alpha_m : Product  Inputs=*/
  alpha_m1 : Product  Inputs=*/
  mNaf : Outport  VectorParamsAs1DForOutWhenUnconnected=off
  wires:
  Gain/1 -> Divide2/2
  Divide/1 -> Add3/1
  Divide5/1 -> Add3/2
  Add/1 -> Divide/1
  Constant/1 -> Add/1
  Divide3/1 -> Divide4/1
  Constant2/1 -> Add1/1
  Constant6/1 -> Divide2/1
  Constant7/1 -> Add4/1
  Add4/1 -> Divide6/1, Gain/1
  Divide6/1 -> Math Function1/1
  Constant10/1 -> Divide6/2
  Divide1/1 -> alpha_m/1
  Integrator Limited/1 -> mNaf/1, Add/2, Divide5/1
  Constant3/1 -> Add2/1
  Constant5/1 -> Divide4/2
  Add1/1 -> Divide3/1, Divide1/2
  Constant1/1 -> Divide1/1
  Add2/1 -> alpha_m/2
  Constant4/1 -> Divide3/2
  Add3/1 -> Integrator Limited/1
  Math Function/1 -> Add2/2
  Divide4/1 -> Math Function/1
  alpha_m/1 -> Divide/2
  Vm/1 -> Add4/2, Add1/2
  Constant8/1 -> Add5/1
  Math Function1/1 -> Add5/2
  Add5/1 -> alpha_m1/2
  alpha_m1/1 -> Divide5/2
  Divide2/1 -> alpha_m1/1

== system NeuralcircuitULInjured08102023_DSD/Neuron 8/Node 7/Naf1/m  ==
  Vm : Inport
  Add{,2..3,5} (4 alike) : Sum  Inputs=+-
  Add1 : Sum
  Add4 : Sum
  Constant : Constant
  Constant1 : Constant  Value=0.186
  Constant10 : Constant  Value=9.16
  Constant2 : Constant  Value=48.4
  Constant3 : Constant
  Constant4 : Constant  Value=-1
  Constant5 : Constant  Value=10.3
  Constant6 : Constant  Value=0.0086
  Constant7 : Constant  Value=42.7
  Constant8 : Constant
  Divide{,1..3,5} (5 alike) : Product  Inputs=**
  Divide4 : Product  Inputs=*/
  Divide6 : Product  Inputs=*/
  Gain : Gain  Gain=-1
  Integrator Limited : Integrator  InitialCondition=mNap0  UpperSaturationLimit=1  LowerSaturationLimit=0
  Math Function : Math  SignedPower=on
  Math Function1 : Math  SignedPower=on
  alpha_m : Product  Inputs=*/
  alpha_m1 : Product  Inputs=*/
  mNap : Outport  VectorParamsAs1DForOutWhenUnconnected=off
  wires:
  Divide/1 -> Add3/1
  Divide5/1 -> Add3/2
  Add/1 -> Divide/1
  Constant/1 -> Add/1
  Divide3/1 -> Divide4/1
  Constant2/1 -> Add1/1
  Constant6/1 -> Divide2/1
  Constant7/1 -> Add4/1
  Add4/1 -> Divide6/1, Gain/1
  Divide6/1 -> Math Function1/1
  Constant10/1 -> Divide6/2
  Divide1/1 -> alpha_m/1
  Integrator Limited/1 -> mNap/1, [mNap], Add/2, Divide5/1
  Constant3/1 -> Add2/1
  Constant5/1 -> Divide4/2
  Add1/1 -> Divide3/1, Divide1/2
  Constant1/1 -> Divide1/1
  Add2/1 -> alpha_m/2
  Constant4/1 -> Divide3/2
  Add3/1 -> Integrator Limited/1
  Math Function/1 -> Add2/2
  Divide4/1 -> Math Function/1
  alpha_m/1 -> Divide/2
  Vm/1 -> Add4/2, Add1/2
  alpha_m1/1 -> Divide5/2
  Divide2/1 -> alpha_m1/1
  Gain/1 -> Divide2/2
  Add5/1 -> alpha_m1/2
  Constant8/1 -> Add5/1
  Math Function1/1 -> Add5/2

== system NeuralcircuitULInjured08102023_DSD/Neuron 8/Node 8/Ks/s  ==
  Vm : Inport
  Add{,2..3,5} (4 alike) : Sum  Inputs=+-
  Add1 : Sum
  Add4 : Sum
  Beta_s : Product  Inputs=*/
  Constant : Constant
  Constant1 : Constant  Value=0.00122
  Constant10 : Constant  Value=21.8
  Constant2 : Constant  Value=19.5
  Constant3 : Constant
  Constant4 : Constant  Value=-1
  Constant5 : Constant  Value=23.6
  Constant6 : Constant  Value=0.000739
  Constant7 : Constant  Value=87.1
  Constant8 : Constant
  Divide{,1..3,5} (5 alike) : Product  Inputs=**
  Divide4 : Product  Inputs=*/
  Divide6 : Product  Inputs=*/
  Gain : Gain  Gain=-1
  Integrator Limited : Integrator  InitialCondition=s0  UpperSaturationLimit=1  LowerSaturationLimit=0
  Math Function : Math  SignedPower=on
  Math Function1 : Math  SignedPower=on
  alpha_m : Product  Inputs=*/
  s : Outport  VectorParamsAs1DForOutWhenUnconnected=off
  wires:
  Divide/1 -> Add3/1
  Divide5/1 -> Add3/2
  Add/1 -> Divide/1
  Constant/1 -> Add/1
  Divide3/1 -> Divide4/1
  Constant2/1 -> Add1/1
  Constant6/1 -> Divide2/1
  Constant7/1 -> Add4/1
  Add4/1 -> Divide6/1, Gain/1
  Divide6/1 -> Math Function1/1
  Constant10/1 -> Divide6/2
  Divide1/1 -> alpha_m/1
  Integrator Limited/1 -> Add/2, Divide5/1, s/1
  Constant3/1 -> Add2/1
  Constant5/1 -> Divide4/2
  Add1/1 -> Divide3/1, Divide1/2
  Constant1/1 -> Divide1/1
  Add2/1 -> alpha_m/2
  Constant4/1 -> Divide3/2
  Add3/1 -> Integrator Limited/1
  Math Function/1 -> Add2/2
  Divide4/1 -> Math Function/1
  alpha_m/1 -> Divide/2
  Vm/1 -> Add4/2, Add1/2
  Gain/1 -> Divide2/2
  Beta_s/1 -> Divide5/2
  Divide2/1 -> Beta_s/1
  Constant8/1 -> Add5/1
  Add5/1 -> Beta_s/2
  Math Function1/1 -> Add5/2

== system NeuralcircuitULInjured08102023_DSD/Neuron 8/Node 8/Naf/h ==
  Vi : Inport
  Add : Sum  Inputs=+-
  Add1 : Sum
  Add2 : Sum  Inputs=+-
  Add3 : Sum  Inputs=+-
  Add4 : Sum
  Add5 : Sum
  Beta_h : Product  Inputs=*/
  Constant : Constant
  Constant1 : Constant  Value=0.0336
  Constant10 : Constant  Value=13.4
  Constant2 : Constant  Value=118
  Constant3 : Constant
  Constant5 : Constant  Value=11
  Constant6 : Constant  Value=2.3
  Constant7 : Constant  Value=35.8
  Constant8 : Constant
  Divide : Product  Inputs=**
  Divide1 : Product  Inputs=**
  Divide4 : Product  Inputs=*/
  Divide5 : Product  Inputs=**
  Divide6 : Product  Inputs=*/
  Gain : Gain  Gain=-1
  Gain1 : Gain  Gain=-1
  Integrator Limited : Integrator  InitialCondition=h0  UpperSaturationLimit=1  LowerSaturationLimit=0
  Math Function : Math  SignedPower=on
  Math Function1 : Math  SignedPower=on
  alpha_h1 : Product  Inputs=*/
  hNaf : Outport  VectorParamsAs1DForOutWhenUnconnected=off
  wires:
  Add5/1 -> Beta_h/2
  Divide/1 -> Add3/1
  Constant6/1 -> Beta_h/1
  Divide5/1 -> Add3/2
  Add/1 -> Divide/1
  Constant/1 -> Add/1
  Add1/1 -> Divide4/1, Gain1/1
  Constant2/1 -> Add1/1
  Constant7/1 -> Add4/1
  Constant8/1 -> Add5/1
  Add4/1 -> Gain/1
  Divide6/1 -> Math Function1/1
  Math Function1/1 -> Add5/2
  Constant10/1 -> Divide6/2
  Constant1/1 -> Divide1/1
  Beta_h/1 -> Divide5/2
  Add3/1 -> Integrator Limited/1
  Divide4/1 -> Math Function/1
  Divide1/1 -> alpha_h1/1
  Vi/1 -> Add4/2, Add1/2
  Gain/1 -> Divide6/1
  Integrator Limited/1 -> hNaf/1, Add/2, Divide5/1
  Gain1/1 -> Divide1/2
  Constant5/1 -> Divide4/2
  Add2/1 -> alpha_h1/2
  Constant3/1 -> Add2/1
  Math Function/1 -> Add2/2
  alpha_h1/1 -> Divide/2

== system NeuralcircuitULInjured08102023_DSD/Neuron 8/Node 8/Naf/m  ==
  Vm : Inport
  Add{,2..3,5} (4 alike) : Sum  Inputs=+-
  Add1 : Sum
  Add4 : Sum
  Constant : Constant
  Constant1 : Constant  Value=1.86
  Constant10 : Constant  Value=9.16
  Constant2 : Constant  Value=25.4
  Constant3 : Constant
  Constant4 : Constant  Value=-1
  Constant5 : Constant  Value=10.3
  Constant6 : Constant  Value=0.086
  Constant7 : Constant  Value=29.7
  Constant8 : Constant
  Divide{,1..3,5} (5 alike) : Product  Inputs=**
  Divide4 : Product  Inputs=*/
  Divide6 : Product  Inputs=*/
  Gain : Gain  Gain=-1
  Integrator Limited : Integrator  InitialCondition=m0  UpperSaturationLimit=1  LowerSaturationLimit=0
  Math Function : Math  SignedPower=on
  Math Function1 : Math  SignedPower=on
  alpha_m : Product  Inputs=*/
  alpha_m1 : Product  Inputs=*/
  mNaf : Outport  VectorParamsAs1DForOutWhenUnconnected=off
  wires:
  Gain/1 -> Divide2/2
  Divide/1 -> Add3/1
  Divide5/1 -> Add3/2
  Add/1 -> Divide/1
  Constant/1 -> Add/1
  Divide3/1 -> Divide4/1
  Constant2/1 -> Add1/1
  Constant6/1 -> Divide2/1
  Constant7/1 -> Add4/1
  Add4/1 -> Divide6/1, Gain/1
  Divide6/1 -> Math Function1/1
  Constant10/1 -> Divide6/2
  Divide1/1 -> alpha_m/1
  Integrator Limited/1 -> mNaf/1, Add/2, Divide5/1
  Constant3/1 -> Add2/1
  Constant5/1 -> Divide4/2
  Add1/1 -> Divide3/1, Divide1/2
  Constant1/1 -> Divide1/1
  Add2/1 -> alpha_m/2
  Constant4/1 -> Divide3/2
  Add3/1 -> Integrator Limited/1
  Math Function/1 -> Add2/2
  Divide4/1 -> Math Function/1
  alpha_m/1 -> Divide/2
  Vm/1 -> Add4/2, Add1/2
  Constant8/1 -> Add5/1
  Math Function1/1 -> Add5/2
  Add5/1 -> alpha_m1/2
  alpha_m1/1 -> Divide5/2
  Divide2/1 -> alpha_m1/1

== system NeuralcircuitULInjured08102023_DSD/Neuron 8/Node 8/Naf1/m  ==
  Vm : Inport
  Add{,2..3,5} (4 alike) : Sum  Inputs=+-
  Add1 : Sum
  Add4 : Sum
  Constant : Constant
  Constant1 : Constant  Value=0.186
  Constant10 : Constant  Value=9.16
  Constant2 : Constant  Value=48.4
  Constant3 : Constant
  Constant4 : Constant  Value=-1
  Constant5 : Constant  Value=10.3
  Constant6 : Constant  Value=0.0086
  Constant7 : Constant  Value=42.7
  Constant8 : Constant
  Divide{,1..3,5} (5 alike) : Product  Inputs=**
  Divide4 : Product  Inputs=*/
  Divide6 : Product  Inputs=*/
  Gain : Gain  Gain=-1
  Integrator Limited : Integrator  InitialCondition=mNap0  UpperSaturationLimit=1  LowerSaturationLimit=0
  Math Function : Math  SignedPower=on
  Math Function1 : Math  SignedPower=on
  alpha_m : Product  Inputs=*/
  alpha_m1 : Product  Inputs=*/
  mNap : Outport  VectorParamsAs1DForOutWhenUnconnected=off
  wires:
  Divide/1 -> Add3/1
  Divide5/1 -> Add3/2
  Add/1 -> Divide/1
  Constant/1 -> Add/1
  Divide3/1 -> Divide4/1
  Constant2/1 -> Add1/1
  Constant6/1 -> Divide2/1
  Constant7/1 -> Add4/1
  Add4/1 -> Divide6/1, Gain/1
  Divide6/1 -> Math Function1/1
  Constant10/1 -> Divide6/2
  Divide1/1 -> alpha_m/1
  Integrator Limited/1 -> mNap/1, [mNap], Add/2, Divide5/1
  Constant3/1 -> Add2/1
  Constant5/1 -> Divide4/2
  Add1/1 -> Divide3/1, Divide1/2
  Constant1/1 -> Divide1/1
  Add2/1 -> alpha_m/2
  Constant4/1 -> Divide3/2
  Add3/1 -> Integrator Limited/1
  Math Function/1 -> Add2/2
  Divide4/1 -> Math Function/1
  alpha_m/1 -> Divide/2
  Vm/1 -> Add4/2, Add1/2
  alpha_m1/1 -> Divide5/2
  Divide2/1 -> alpha_m1/1
  Gain/1 -> Divide2/2
  Add5/1 -> alpha_m1/2
  Constant8/1 -> Add5/1
  Math Function1/1 -> Add5/2

== system NeuralcircuitULInjured08102023_DSD/Neuron 8/Node 9/Ks/s  ==
  Vm : Inport
  Add{,2..3,5} (4 alike) : Sum  Inputs=+-
  Add1 : Sum
  Add4 : Sum
  Beta_s : Product  Inputs=*/
  Constant : Constant
  Constant1 : Constant  Value=0.00122
  Constant10 : Constant  Value=21.8
  Constant2 : Constant  Value=19.5
  Constant3 : Constant
  Constant4 : Constant  Value=-1
  Constant5 : Constant  Value=23.6
  Constant6 : Constant  Value=0.000739
  Constant7 : Constant  Value=87.1
  Constant8 : Constant
  Divide{,1..3,5} (5 alike) : Product  Inputs=**
  Divide4 : Product  Inputs=*/
  Divide6 : Product  Inputs=*/
  Gain : Gain  Gain=-1
  Integrator Limited : Integrator  InitialCondition=s0  UpperSaturationLimit=1  LowerSaturationLimit=0
  Math Function : Math  SignedPower=on
  Math Function1 : Math  SignedPower=on
  alpha_m : Product  Inputs=*/
  s : Outport  VectorParamsAs1DForOutWhenUnconnected=off
  wires:
  Divide/1 -> Add3/1
  Divide5/1 -> Add3/2
  Add/1 -> Divide/1
  Constant/1 -> Add/1
  Divide3/1 -> Divide4/1
  Constant2/1 -> Add1/1
  Constant6/1 -> Divide2/1
  Constant7/1 -> Add4/1
  Add4/1 -> Divide6/1, Gain/1
  Divide6/1 -> Math Function1/1
  Constant10/1 -> Divide6/2
  Divide1/1 -> alpha_m/1
  Integrator Limited/1 -> Add/2, Divide5/1, s/1
  Constant3/1 -> Add2/1
  Constant5/1 -> Divide4/2
  Add1/1 -> Divide3/1, Divide1/2
  Constant1/1 -> Divide1/1
  Add2/1 -> alpha_m/2
  Constant4/1 -> Divide3/2
  Add3/1 -> Integrator Limited/1
  Math Function/1 -> Add2/2
  Divide4/1 -> Math Function/1
  alpha_m/1 -> Divide/2
  Vm/1 -> Add4/2, Add1/2
  Gain/1 -> Divide2/2
  Beta_s/1 -> Divide5/2
  Divide2/1 -> Beta_s/1
  Constant8/1 -> Add5/1
  Add5/1 -> Beta_s/2
  Math Function1/1 -> Add5/2

== system NeuralcircuitULInjured08102023_DSD/Neuron 8/Node 9/Naf/h ==
  Vi : Inport
  Add : Sum  Inputs=+-
  Add1 : Sum
  Add2 : Sum  Inputs=+-
  Add3 : Sum  Inputs=+-
  Add4 : Sum
  Add5 : Sum
  Beta_h : Product  Inputs=*/
  Constant : Constant
  Constant1 : Constant  Value=0.0336
  Constant10 : Constant  Value=13.4
  Constant2 : Constant  Value=118
  Constant3 : Constant
  Constant5 : Constant  Value=11
  Constant6 : Constant  Value=2.3
  Constant7 : Constant  Value=35.8
  Constant8 : Constant
  Divide : Product  Inputs=**
  Divide1 : Product  Inputs=**
  Divide4 : Product  Inputs=*/
  Divide5 : Product  Inputs=**
  Divide6 : Product  Inputs=*/
  Gain : Gain  Gain=-1
  Gain1 : Gain  Gain=-1
  Integrator Limited : Integrator  InitialCondition=h0  UpperSaturationLimit=1  LowerSaturationLimit=0
  Math Function : Math  SignedPower=on
  Math Function1 : Math  SignedPower=on
  alpha_h1 : Product  Inputs=*/
  hNaf : Outport  VectorParamsAs1DForOutWhenUnconnected=off
  wires:
  Add5/1 -> Beta_h/2
  Divide/1 -> Add3/1
  Constant6/1 -> Beta_h/1
  Divide5/1 -> Add3/2
  Add/1 -> Divide/1
  Constant/1 -> Add/1
  Add1/1 -> Divide4/1, Gain1/1
  Constant2/1 -> Add1/1
  Constant7/1 -> Add4/1
  Constant8/1 -> Add5/1
  Add4/1 -> Gain/1
  Divide6/1 -> Math Function1/1
  Math Function1/1 -> Add5/2
  Constant10/1 -> Divide6/2
  Constant1/1 -> Divide1/1
  Beta_h/1 -> Divide5/2
  Add3/1 -> Integrator Limited/1
  Divide4/1 -> Math Function/1
  Divide1/1 -> alpha_h1/1
  Vi/1 -> Add4/2, Add1/2
  Gain/1 -> Divide6/1
  Integrator Limited/1 -> hNaf/1, Add/2, Divide5/1
  Gain1/1 -> Divide1/2
  Constant5/1 -> Divide4/2
  Add2/1 -> alpha_h1/2
  Constant3/1 -> Add2/1
  Math Function/1 -> Add2/2
  alpha_h1/1 -> Divide/2

== system NeuralcircuitULInjured08102023_DSD/Neuron 8/Node 9/Naf/m  ==
  Vm : Inport
  Add{,2..3,5} (4 alike) : Sum  Inputs=+-
  Add1 : Sum
  Add4 : Sum
  Constant : Constant
  Constant1 : Constant  Value=1.86
  Constant10 : Constant  Value=9.16
  Constant2 : Constant  Value=25.4
  Constant3 : Constant
  Constant4 : Constant  Value=-1
  Constant5 : Constant  Value=10.3
  Constant6 : Constant  Value=0.086
  Constant7 : Constant  Value=29.7
  Constant8 : Constant
  Divide{,1..3,5} (5 alike) : Product  Inputs=**
  Divide4 : Product  Inputs=*/
  Divide6 : Product  Inputs=*/
  Gain : Gain  Gain=-1
  Integrator Limited : Integrator  InitialCondition=m0  UpperSaturationLimit=1  LowerSaturationLimit=0
  Math Function : Math  SignedPower=on
  Math Function1 : Math  SignedPower=on
  alpha_m : Product  Inputs=*/
  alpha_m1 : Product  Inputs=*/
  mNaf : Outport  VectorParamsAs1DForOutWhenUnconnected=off
  wires:
  Gain/1 -> Divide2/2
  Divide/1 -> Add3/1
  Divide5/1 -> Add3/2
  Add/1 -> Divide/1
  Constant/1 -> Add/1
  Divide3/1 -> Divide4/1
  Constant2/1 -> Add1/1
  Constant6/1 -> Divide2/1
  Constant7/1 -> Add4/1
  Add4/1 -> Divide6/1, Gain/1
  Divide6/1 -> Math Function1/1
  Constant10/1 -> Divide6/2
  Divide1/1 -> alpha_m/1
  Integrator Limited/1 -> mNaf/1, Add/2, Divide5/1
  Constant3/1 -> Add2/1
  Constant5/1 -> Divide4/2
  Add1/1 -> Divide3/1, Divide1/2
  Constant1/1 -> Divide1/1
  Add2/1 -> alpha_m/2
  Constant4/1 -> Divide3/2
  Add3/1 -> Integrator Limited/1
  Math Function/1 -> Add2/2
  Divide4/1 -> Math Function/1
  alpha_m/1 -> Divide/2
  Vm/1 -> Add4/2, Add1/2
  Constant8/1 -> Add5/1
  Math Function1/1 -> Add5/2
  Add5/1 -> alpha_m1/2
  alpha_m1/1 -> Divide5/2
  Divide2/1 -> alpha_m1/1
